simulink model "Punto7"  (R2025b)
settings: Solver=ode45  StartTime=0.0  StopTime=10  MaxStep=0.01  RelTol=1e-4
libraries: fuzblock x1, simulink x1
settings Model: Creator=Estudiantes

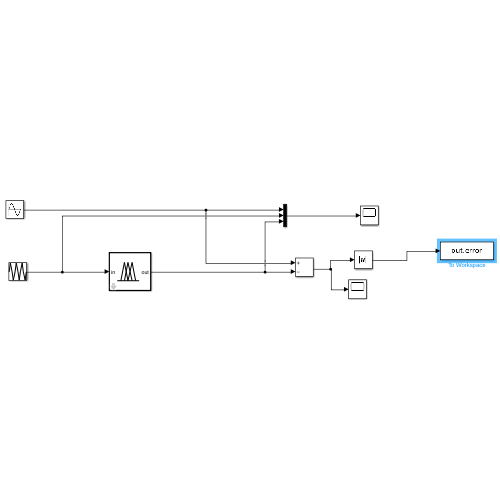
[thumbnail: Simulink's stored preview of the top-level diagram]
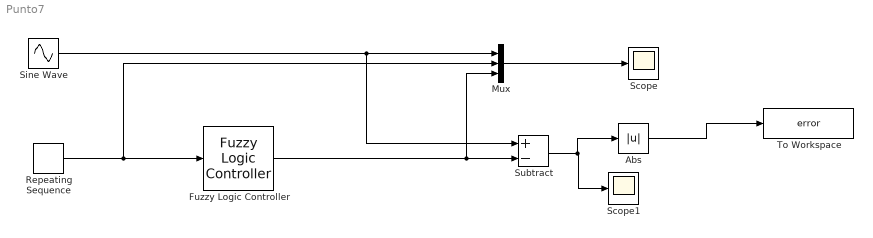
== system Punto7 ==
  Abs : Abs  SaturateOnIntegerOverflow=off
  Fuzzy Logic Controller : fuzblock/Fuzzy Logic  Controller  FIS='triangularA2seno_11mf.fis'  OutputSampleNumber=101  DataType=double  UseLookupTable=off  NumBreakpoints=10  FuzzifiedInputs=off  RuleFiringStrengths=off  RuleOutputs=off  AggregatedOutputs=off  SimulateUsing=Interpreted execution  OutOfRangeInputValueMessage=warning  NoRuleFiredMessage=warning  EmptyOutputFuzzySetMessage=warning
  Mux : Mux  Inputs=3
  Repeating Sequence : simulink/Sources/Repeating Sequence  rep_seq_t=[0 0.5 1 1.5 2]  rep_seq_y=[0 0.5 0 -0.5 0]
  Scope : Scope
      settings: ActiveDisplayYMinimum=-0.49469919787926719  ActiveDisplayYMaximum=0.63908765019329539
  Scope1 : Scope
      settings: ActiveDisplayYMinimum=-0.061071935509620895  ActiveDisplayYMaximum=0.061071935509621228
  Sine Wave : Sin  Amplitude=0.5  Frequency=pi  SampleTime=0
  Subtract : Sum  Inputs=+-
  To Workspace : ToWorkspace  VariableName=error  SampleTime=-1
  wires:
  Sine Wave/1 -> Subtract/1, Mux/1
  Repeating Sequence/1 -> Mux/2, Fuzzy Logic Controller/1
  Fuzzy Logic Controller/1 -> Mux/3, Subtract/2
  Subtract/1 -> Abs/1, Scope1/1
  Mux/1 -> Scope/1
  Abs/1 -> To Workspace/1
